simulink model "Demo_Intersection_cs"  (Simulink 7.6)
settings: Solver=FixedStepDiscrete  SolverMode=SingleTasking  StartTime=0.0  StopTime=13  FixedStep=1/20  RelTol=1e-3
PreLoadFcn:
  | check_NUTS_defined
  | model_closed = 0;
  | assignin('base',['model_closed_' bdroot],false);
InitFcn:
  | PreScanExperimentInitFcn(bdroot)
StopFcn:
  | PreScanExperimentStopFcn(bdroot);
  | 
undefined symbols (not defined in the file or in its folder): DiscIntNeverNeededParam
libraries: PreScanSimulinkLibrary x32, PreScanUsefulBlocks x8, simulink_extras x3
(part 2 of 5)

== system Demo_Intersection_cs/STATE_Toyota_Yaris_1 ==
  State : Inport  SampleTime=TimeStep
  Acceleration : Subsystem  mask(ToSensorWorld){PortName=Acceleration_Toyota_Yaris_1, PortIndex=21, PortWidth=3, TimeStep=1/20}
      mask prompts: PortName "Port Name [-]"; PortIndex "Index [-]"; PortWidth "Port Dimensions [-]"; TimeStep "Upload Period [s]"
      mask help: Sends signal(s) from Simulink to the Sensor World
      mask Help:
      | Sends signal(s) from Simulink to the Sensor World.
      | 
      | - Port Name [-]: specifies the name of the output terminal of the Simulink block.
      | - Index [-]: specifies the start position in the output vector sent to the Sensor World
      | - Port dimensions [-]: specifies the width (number of scalars) of the output port
      | - Upload period [s]: specifies the upload period (in seconds) of the port.
      mask Display: port_label('input', 1, PortName)
  Demux : Demux  Outputs=5
  Position : Subsystem  mask(ToSensorWorld){PortName=Position_Toyota_Yaris_1, PortIndex=15, PortWidth=3, TimeStep=1/20}
      mask prompts: PortName "Port Name [-]"; PortIndex "Index [-]"; PortWidth "Port Dimensions [-]"; TimeStep "Upload Period [s]"
      mask help: Sends signal(s) from Simulink to the Sensor World
      mask Help:
      | Sends signal(s) from Simulink to the Sensor World.
      | 
      | - Port Name [-]: specifies the name of the output terminal of the Simulink block.
      | - Index [-]: specifies the start position in the output vector sent to the Sensor World
      | - Port dimensions [-]: specifies the width (number of scalars) of the output port
      | - Upload period [s]: specifies the upload period (in seconds) of the port.
      mask Display: port_label('input', 1, PortName)
  RPY : Subsystem  mask(ToSensorWorld){PortName=RPY_Toyota_Yaris_1, PortIndex=24, PortWidth=3, TimeStep=1/20}
      mask prompts: PortName "Port Name [-]"; PortIndex "Index [-]"; PortWidth "Port Dimensions [-]"; TimeStep "Upload Period [s]"
      mask help: Sends signal(s) from Simulink to the Sensor World
      mask Help:
      | Sends signal(s) from Simulink to the Sensor World.
      | 
      | - Port Name [-]: specifies the name of the output terminal of the Simulink block.
      | - Index [-]: specifies the start position in the output vector sent to the Sensor World
      | - Port dimensions [-]: specifies the width (number of scalars) of the output port
      | - Upload period [s]: specifies the upload period (in seconds) of the port.
      mask Display: port_label('input', 1, PortName)
  Velocity : Subsystem  mask(ToSensorWorld){PortName=Velocity_Toyota_Yaris_1, PortIndex=18, PortWidth=3, TimeStep=1/20}
      mask prompts: PortName "Port Name [-]"; PortIndex "Index [-]"; PortWidth "Port Dimensions [-]"; TimeStep "Upload Period [s]"
      mask help: Sends signal(s) from Simulink to the Sensor World
      mask Help:
      | Sends signal(s) from Simulink to the Sensor World.
      | 
      | - Port Name [-]: specifies the name of the output terminal of the Simulink block.
      | - Index [-]: specifies the start position in the output vector sent to the Sensor World
      | - Port dimensions [-]: specifies the width (number of scalars) of the output port
      | - Upload period [s]: specifies the upload period (in seconds) of the port.
      mask Display: port_label('input', 1, PortName)
  iniBODYAngles wrtVEH [rad] : Constant  Value=[Roll0 Pitch0 0]  SampleTime=TimeStep
  iniVEHAngles wrtGLOB [rad] : Constant  Value=[0 0 Yaw0]  SampleTime=TimeStep
  iniVEHposition wrtGLOB [m] : Constant  Value=[x0 y0 z0]  SampleTime=TimeStep
  state2FullState : PreScanSimulinkLibrary/state2FullState  SystemSampleTime=-1
  velRPY : Subsystem  mask(ToSensorWorld){PortName=velRPY_Toyota_Yaris_1, PortIndex=27, PortWidth=3, TimeStep=1/20}
      mask prompts: PortName "Port Name [-]"; PortIndex "Index [-]"; PortWidth "Port Dimensions [-]"; TimeStep "Upload Period [s]"
      mask help: Sends signal(s) from Simulink to the Sensor World
      mask Help:
      | Sends signal(s) from Simulink to the Sensor World.
      | 
      | - Port Name [-]: specifies the name of the output terminal of the Simulink block.
      | - Index [-]: specifies the start position in the output vector sent to the Sensor World
      | - Port dimensions [-]: specifies the width (number of scalars) of the output port
      | - Upload period [s]: specifies the upload period (in seconds) of the port.
      mask Display: port_label('input', 1, PortName)
  wires:
  Demux/5 -> velRPY/1(Y)
  Demux/4 -> RPY/1(Y)
  Demux/3 -> Acceleration/1(Y)
  Demux/2 -> Velocity/1(Y)
  Demux/1 -> Position/1(Y)
  State/1 -> state2FullState/1
  state2FullState/1 -> Demux/1
  iniVEHposition wrtGLOB [m]/1 -> state2FullState/2
  iniBODYAngles wrtVEH [rad]/1 -> state2FullState/3
  iniVEHAngles wrtGLOB [rad]/1 -> state2FullState/4

== system Demo_Intersection_cs/SetActuators ==
  Bus Creator : BusCreator  Inputs=1
  Data Store Read : DataStoreRead  DataStoreName=SimCoreActuators  SampleTime=TimeStep
  SendActuators : M-S-Function  FunctionName=SendActuatorsBlock  Parameters=TimeStep NrOfActuators
  dummy : Outport
  tag scope: SimCoreInfo=global
  wires:
  Bus Creator/1 -> [SimCoreInfo]  "SimCore"
  SendActuators/2 -> Bus Creator/1  "ComputationTime[s]"
  SendActuators/1 -> dummy/1
  Data Store Read/1 -> SendActuators/1

== system Demo_Intersection_cs/SimCoreInfo ==
  Bus Selector : BusSelector  OutputSignals=ComputationTime[s]
  Time : Scope
      settings: TimeRange=10  YMin=0  YMax=0.5  SaveName=ComputationTime
  wires:
  Bus Selector/1 -> Time/1  "<ComputationTime[s]>"
  [SimCoreInfo] -> Bus Selector/1

== system Demo_Intersection_cs/Toyota_Previa_1 ==
  SELF_Toyota_Previa_1 : Inport  Tag=SELFInport
  Antenna_Tx_3_BusAssignment : BusAssignment  Tag=BusAntennaT  AssignedSignals=Intention
  Antenna_Tx_3_Mux : Subsystem  Tag=MuxAntennaT  mask(PreScan Mux Block:){Channel=1, TimeStep=1/20}
      mask prompts: TimeStep "Time Step [s]"
      settings: DeleteFcn=PreScanBlockDeleteFcn;
      mask Display:
      | fprintf('Channel: %d',Channel)
      | port_label('input', 1, 'Warning signal ID')
      | port_label('input', 2, 'Maneuvre ID')
      | port_label('input', 3, 'Vehicle Type')
      | port_label('input', 4, 'Braking Capacity')
      | port_label('input', 5, 'Vehicle Size')
      | port_label('input', 6, 'spare')
  Constant1 : Constant  Value=2
  Ground_{1..5} (5 alike) : Ground
  SELF_Demux : Subsystem  Tag=DemuxSELF
      settings: DeleteFcn=PreScanBlockDeleteFcn;
      mask Type: PreScan Demux Block:
      mask Display:
      | port_label('output',1,'x [m]')
      | port_label('output',2,'y [m]')
      | port_label('output',3,'z [m]','texmode','on')
      | port_label('output',4,'Rotx [deg]','texmode','on')
      | port_label('output',5,'Roty [deg]','texmode','on')
      | port_label('output',6,'Rotz [deg]','texmode','on')
      | port_label('output',7,'GPS lat [deg]','texmode','on')
      | port_label('output',8,'GPS long [deg]','texmode','on')
      | port_label('output',9,'GPS alt [m]','texmode','on')
      | port_label('output',10,'Velocity [m/s]')
      | port_label('output',11,'Heading [deg]')
      | port_label('output',12,'Yaw rate [deg/s]')
  Sum : Sum  Inputs=|++
  Terminator_{1..12} (12 alike) : Terminator
  Trajectories : Subsystem  Tag=Trajectories
      mask Display: image(imread('Trajectory.png'));
  STATE_Toyota_Previa_1 : Outport  Tag=StateOutport
  Antenna_Tx_3 : Outport  Tag=AntennaTOutport  Port=2
  wires:
  Constant1/1 -> Sum/2
  [Lane3_Intention] -> Sum/1
  SELF_Toyota_Previa_1/1 -> SELF_Demux/1(SELF)
  Antenna_Tx_3_Mux/2(Out2) -> [Antenna_Tx_3]
  [Antenna_Tx_3] -> Antenna_Tx_3_BusAssignment/1
  Antenna_Tx_3_BusAssignment/1 -> Antenna_Tx_3_Mux/6(spare)
  Antenna_Tx_3_Mux/1(Out1) -> Antenna_Tx_3/1
  Trajectories/1(State) -> STATE_Toyota_Previa_1/1
  Sum/1 -> Trajectories/1(In1)
  [Lane3_Intention] -> Antenna_Tx_3_BusAssignment/2
  Ground_1/1 -> Antenna_Tx_3_Mux/1(warning_signal_id)
  Ground_2/1 -> Antenna_Tx_3_Mux/2(maneuvre_id)
  Ground_3/1 -> Antenna_Tx_3_Mux/3(vehicle_type)
  Ground_4/1 -> Antenna_Tx_3_Mux/4(brakingcapacity)
  Ground_5/1 -> Antenna_Tx_3_Mux/5(vehicle_size)
  SELF_Demux/1(x [m]) -> Terminator_1/1
  SELF_Demux/2(y [m]) -> Terminator_2/1
  SELF_Demux/3(z [m]) -> Terminator_3/1
  SELF_Demux/4(rotx [deg]) -> Terminator_4/1
  SELF_Demux/5(roty [deg]) -> Terminator_5/1
  SELF_Demux/6(rotz [deg]) -> Terminator_6/1
  SELF_Demux/7(GPS lat [deg]) -> Terminator_7/1
  SELF_Demux/8(GPS long [deg]) -> Terminator_8/1
  SELF_Demux/9(GPS alt [m]) -> Terminator_9/1
  SELF_Demux/10(velocity [m/s]) -> Terminator_10/1
  SELF_Demux/11(heading [deg]) -> Terminator_11/1
  SELF_Demux/12(yaw rate [deg/s]) -> Terminator_12/1

== system Demo_Intersection_cs/Toyota_Yaris_1 ==
  SELF_Toyota_Yaris_1 : Inport  Tag=SELFInport
  Antenna_Tx_2_BusAssignment : BusAssignment  Tag=BusAntennaT  AssignedSignals=Intention
  Antenna_Tx_2_Mux : Subsystem  Tag=MuxAntennaT  mask(PreScan Mux Block:){Channel=1, TimeStep=1/20}
      mask prompts: TimeStep "Time Step [s]"
      settings: DeleteFcn=PreScanBlockDeleteFcn;
      mask Display:
      | fprintf('Channel: %d',Channel)
      | port_label('input', 1, 'Warning signal ID')
      | port_label('input', 2, 'Maneuvre ID')
      | port_label('input', 3, 'Vehicle Type')
      | port_label('input', 4, 'Braking Capacity')
      | port_label('input', 5, 'Vehicle Size')
      | port_label('input', 6, 'spare')
  Constant1 : Constant  Value=2
  Ground_{1..5} (5 alike) : Ground
  SELF_Demux : Subsystem  Tag=DemuxSELF
      settings: DeleteFcn=PreScanBlockDeleteFcn;
      mask Type: PreScan Demux Block:
      mask Display:
      | port_label('output',1,'x [m]')
      | port_label('output',2,'y [m]')
      | port_label('output',3,'z [m]','texmode','on')
      | port_label('output',4,'Rotx [deg]','texmode','on')
      | port_label('output',5,'Roty [deg]','texmode','on')
      | port_label('output',6,'Rotz [deg]','texmode','on')
      | port_label('output',7,'GPS lat [deg]','texmode','on')
      | port_label('output',8,'GPS long [deg]','texmode','on')
      | port_label('output',9,'GPS alt [m]','texmode','on')
      | port_label('output',10,'Velocity [m/s]')
      | port_label('output',11,'Heading [deg]')
      | port_label('output',12,'Yaw rate [deg/s]')
  Sum : Sum  Inputs=|++
  Terminator_{1..12} (12 alike) : Terminator
  Trajectories : Subsystem  Tag=Trajectories
      mask Display: image(imread('Trajectory.png'));
  STATE_Toyota_Yaris_1 : Outport  Tag=StateOutport
  Antenna_Tx_2 : Outport  Tag=AntennaTOutport  Port=2
  wires:
  Constant1/1 -> Sum/2
  [Lane2_Intention] -> Sum/1
  SELF_Toyota_Yaris_1/1 -> SELF_Demux/1(SELF)
  Antenna_Tx_2_Mux/2(Out2) -> [Antenna_Tx_2]
  [Antenna_Tx_2] -> Antenna_Tx_2_BusAssignment/1
  Antenna_Tx_2_BusAssignment/1 -> Antenna_Tx_2_Mux/6(spare)
  Antenna_Tx_2_Mux/1(Out1) -> Antenna_Tx_2/1
  Trajectories/1(State) -> STATE_Toyota_Yaris_1/1
  Sum/1 -> Trajectories/1(In1)
  [Lane2_Intention] -> Antenna_Tx_2_BusAssignment/2
  Ground_1/1 -> Antenna_Tx_2_Mux/1(warning_signal_id)
  Ground_2/1 -> Antenna_Tx_2_Mux/2(maneuvre_id)
  Ground_3/1 -> Antenna_Tx_2_Mux/3(vehicle_type)
  Ground_4/1 -> Antenna_Tx_2_Mux/4(brakingcapacity)
  Ground_5/1 -> Antenna_Tx_2_Mux/5(vehicle_size)
  SELF_Demux/1(x [m]) -> Terminator_1/1
  SELF_Demux/2(y [m]) -> Terminator_2/1
  SELF_Demux/3(z [m]) -> Terminator_3/1
  SELF_Demux/4(rotx [deg]) -> Terminator_4/1
  SELF_Demux/5(roty [deg]) -> Terminator_5/1
  SELF_Demux/6(rotz [deg]) -> Terminator_6/1
  SELF_Demux/7(GPS lat [deg]) -> Terminator_7/1
  SELF_Demux/8(GPS long [deg]) -> Terminator_8/1
  SELF_Demux/9(GPS alt [m]) -> Terminator_9/1
  SELF_Demux/10(velocity [m/s]) -> Terminator_10/1
  SELF_Demux/11(heading [deg]) -> Terminator_11/1
  SELF_Demux/12(yaw rate [deg/s]) -> Terminator_12/1

== system Demo_Intersection_cs/Mazda_RX8_1/Antenna_Rx_1_Demux ==
  AntennaR : Inport
  Bus Creator : BusCreator  Inputs=200
  Demux : Demux  Outputs=228
  Demux1 : Demux  Outputs=3
  Mux : Mux  Inputs=3
  Reorder : Subsystem  mask(Output reorder block){NrOfOutputs=228, NrOfObjects=3}
      mask prompts: NrOfOutputs "Number Of Outputs [-]"; NrOfObjects "Number Of Objects [-]"
      mask help: Change output order from object based to output type based
      mask init:
      | InputPortWidth=NrOfObjects*NrOfOutputs;
      | Input=1:InputPortWidth;
      | ReshapedInput=reshape(Input,NrOfOutputs,NrOfObjects);
      | TransposedReshapedInput=transpose(ReshapedInput);
      | Elements=reshape(TransposedReshapedInput,length(Input),1);
  Terminator_{9..12,17..18,20..23,25..30} (16 alike) : Terminator
  compas converter : Subsystem
  xyz2GPS : PreScanUsefulBlocks/xyz2GPS  CoordinateCount=3  GPS_base=[0.000000 0.000000 0.000]
  Vehicle_ID : Outport
  GPS_pos_lat_[deg] : Outport  Port=2
  GPS_pos_long_[deg] : Outport  Port=3
  GPS_pos_alt_[m] : Outport  Port=4
  Velocity_[m/s] : Outport  Port=5
  Acceleration_[m/s2] : Outport  Port=6
  Heading [deg] : Outport  Port=7
  warning_signal_id : Outport  Port=8
  maneuvre_id : Outport  Port=9
  vehicle_type : Outport  Port=10
  brakingcapacity : Outport  Port=11
  vehicle_size : Outport  Port=12
  spare : Outport  Port=13
  wires:
  Bus Creator/1 -> spare/1
  compas converter/1(heading [deg]) -> Heading [deg]/1
  Demux/1 -> Vehicle_ID/1
  Demux/2 -> Terminator_9/1
  Demux/3 -> Terminator_10/1
  Demux/4 -> Terminator_11/1
  Demux/5 -> Terminator_12/1
  Demux/6 -> Mux/1  "pos_x"
  Demux/7 -> Mux/2  "pos_y"
  Demux/8 -> Mux/3  "pos_z"
  Demux/10 -> Terminator_17/1
  Demux/11 -> Terminator_18/1
  Demux/12 -> Acceleration_[m/s2]/1
  Demux/13 -> Terminator_20/1
  Demux/14 -> Terminator_21/1
  Demux/15 -> Terminator_22/1
  Demux/16 -> Terminator_23/1
  Demux/17 -> compas converter/1(rotz [rad])
  Demux/18 -> Terminator_25/1
  Demux/19 -> Terminator_26/1
  Demux/20 -> Terminator_27/1
  Demux/21 -> Terminator_28/1
  Demux/22 -> Terminator_29/1
  Demux/23 -> Terminator_30/1
  Demux/9 -> Velocity_[m/s]/1
  Demux/24 -> warning_signal_id/1
  Demux/25 -> maneuvre_id/1
  Demux/26 -> vehicle_type/1
  Demux/27 -> brakingcapacity/1
  Demux/28 -> vehicle_size/1
  xyz2GPS/1 -> Demux1/1
  Demux1/1 -> GPS_pos_lat_[deg]/1
  Demux1/2 -> GPS_pos_long_[deg]/1
  Demux1/3 -> GPS_pos_alt_[m]/1
  Mux/1 -> xyz2GPS/1
  Reorder/1(Out) -> Demux/1
  AntennaR/1 -> Reorder/1(In)
  Demux/29 -> Bus Creator/1  "Intention"
  Demux/30 -> Bus Creator/2  "spare_2"
  Demux/31 -> Bus Creator/3  "spare_3"
  Demux/32 -> Bus Creator/4  "spare_4"
  Demux/33 -> Bus Creator/5  "spare_5"
  Demux/34 -> Bus Creator/6  "spare_6"
  Demux/35 -> Bus Creator/7  "spare_7"
  Demux/36 -> Bus Creator/8  "spare_8"
  Demux/37 -> Bus Creator/9  "spare_9"
  Demux/38 -> Bus Creator/10  "spare_10"
  Demux/39 -> Bus Creator/11  "spare_11"
  Demux/40 -> Bus Creator/12  "spare_12"
  Demux/41 -> Bus Creator/13  "spare_13"
  Demux/42 -> Bus Creator/14  "spare_14"
  Demux/43 -> Bus Creator/15  "spare_15"
  Demux/44 -> Bus Creator/16  "spare_16"
  Demux/45 -> Bus Creator/17  "spare_17"
  Demux/46 -> Bus Creator/18  "spare_18"
  Demux/47 -> Bus Creator/19  "spare_19"
  Demux/48 -> Bus Creator/20  "spare_20"
  Demux/49 -> Bus Creator/21  "spare_21"
  Demux/50 -> Bus Creator/22  "spare_22"
  Demux/51 -> Bus Creator/23  "spare_23"
  Demux/52 -> Bus Creator/24  "spare_24"
  Demux/53 -> Bus Creator/25  "spare_25"
  Demux/54 -> Bus Creator/26  "spare_26"
  Demux/55 -> Bus Creator/27  "spare_27"
  Demux/56 -> Bus Creator/28  "spare_28"
  Demux/57 -> Bus Creator/29  "spare_29"
  Demux/58 -> Bus Creator/30  "spare_30"
  Demux/59 -> Bus Creator/31  "spare_31"
  Demux/60 -> Bus Creator/32  "spare_32"
  Demux/61 -> Bus Creator/33  "spare_33"
  Demux/62 -> Bus Creator/34  "spare_34"
  Demux/63 -> Bus Creator/35  "spare_35"
  Demux/64 -> Bus Creator/36  "spare_36"
  Demux/65 -> Bus Creator/37  "spare_37"
  Demux/66 -> Bus Creator/38  "spare_38"
  Demux/67 -> Bus Creator/39  "spare_39"
  Demux/68 -> Bus Creator/40  "spare_40"
  Demux/69 -> Bus Creator/41  "spare_41"
  Demux/70 -> Bus Creator/42  "spare_42"
  Demux/71 -> Bus Creator/43  "spare_43"
  Demux/72 -> Bus Creator/44  "spare_44"
  Demux/73 -> Bus Creator/45  "spare_45"
  Demux/74 -> Bus Creator/46  "spare_46"
  Demux/75 -> Bus Creator/47  "spare_47"
  Demux/76 -> Bus Creator/48  "spare_48"
  Demux/77 -> Bus Creator/49  "spare_49"
  Demux/78 -> Bus Creator/50  "spare_50"
  Demux/79 -> Bus Creator/51  "spare_51"
  Demux/80 -> Bus Creator/52  "spare_52"
  Demux/81 -> Bus Creator/53  "spare_53"
  Demux/82 -> Bus Creator/54  "spare_54"
  Demux/83 -> Bus Creator/55  "spare_55"
  Demux/84 -> Bus Creator/56  "spare_56"
  Demux/85 -> Bus Creator/57  "spare_57"
  Demux/86 -> Bus Creator/58  "spare_58"
  Demux/87 -> Bus Creator/59  "spare_59"
  Demux/88 -> Bus Creator/60  "spare_60"
  Demux/89 -> Bus Creator/61  "spare_61"
  Demux/90 -> Bus Creator/62  "spare_62"
  Demux/91 -> Bus Creator/63  "spare_63"
  Demux/92 -> Bus Creator/64  "spare_64"
  Demux/93 -> Bus Creator/65  "spare_65"
  Demux/94 -> Bus Creator/66  "spare_66"
  Demux/95 -> Bus Creator/67  "spare_67"
  Demux/96 -> Bus Creator/68  "spare_68"
  Demux/97 -> Bus Creator/69  "spare_69"
  Demux/98 -> Bus Creator/70  "spare_70"
  Demux/99 -> Bus Creator/71  "spare_71"
  Demux/100 -> Bus Creator/72  "spare_72"
  Demux/101 -> Bus Creator/73  "spare_73"
  Demux/102 -> Bus Creator/74  "spare_74"
  Demux/103 -> Bus Creator/75  "spare_75"
  Demux/104 -> Bus Creator/76  "spare_76"
  Demux/105 -> Bus Creator/77  "spare_77"
  Demux/106 -> Bus Creator/78  "spare_78"
  Demux/107 -> Bus Creator/79  "spare_79"
  Demux/108 -> Bus Creator/80  "spare_80"
  Demux/109 -> Bus Creator/81  "spare_81"
  Demux/110 -> Bus Creator/82  "spare_82"
  Demux/111 -> Bus Creator/83  "spare_83"
  Demux/112 -> Bus Creator/84  "spare_84"
  Demux/113 -> Bus Creator/85  "spare_85"
  Demux/114 -> Bus Creator/86  "spare_86"
  Demux/115 -> Bus Creator/87  "spare_87"
  Demux/116 -> Bus Creator/88  "spare_88"
  Demux/117 -> Bus Creator/89  "spare_89"
  Demux/118 -> Bus Creator/90  "spare_90"
  Demux/119 -> Bus Creator/91  "spare_91"
  Demux/120 -> Bus Creator/92  "spare_92"
  Demux/121 -> Bus Creator/93  "spare_93"
  Demux/122 -> Bus Creator/94  "spare_94"
  Demux/123 -> Bus Creator/95  "spare_95"
  Demux/124 -> Bus Creator/96  "spare_96"
  Demux/125 -> Bus Creator/97  "spare_97"
  Demux/126 -> Bus Creator/98  "spare_98"
  Demux/127 -> Bus Creator/99  "spare_99"
  Demux/128 -> Bus Creator/100  "spare_100"
  Demux/129 -> Bus Creator/101  "spare_101"
  Demux/130 -> Bus Creator/102  "spare_102"
  Demux/131 -> Bus Creator/103  "spare_103"
  Demux/132 -> Bus Creator/104  "spare_104"
  Demux/133 -> Bus Creator/105  "spare_105"
  Demux/134 -> Bus Creator/106  "spare_106"
  Demux/135 -> Bus Creator/107  "spare_107"
  Demux/136 -> Bus Creator/108  "spare_108"
  Demux/137 -> Bus Creator/109  "spare_109"
  Demux/138 -> Bus Creator/110  "spare_110"
  Demux/139 -> Bus Creator/111  "spare_111"
  Demux/140 -> Bus Creator/112  "spare_112"
  Demux/141 -> Bus Creator/113  "spare_113"
  Demux/142 -> Bus Creator/114  "spare_114"
  Demux/143 -> Bus Creator/115  "spare_115"
  Demux/144 -> Bus Creator/116  "spare_116"
  Demux/145 -> Bus Creator/117  "spare_117"
  Demux/146 -> Bus Creator/118  "spare_118"
  Demux/147 -> Bus Creator/119  "spare_119"
  Demux/148 -> Bus Creator/120  "spare_120"
  Demux/149 -> Bus Creator/121  "spare_121"
  Demux/150 -> Bus Creator/122  "spare_122"
  Demux/151 -> Bus Creator/123  "spare_123"
  Demux/152 -> Bus Creator/124  "spare_124"
  Demux/153 -> Bus Creator/125  "spare_125"
  Demux/154 -> Bus Creator/126  "spare_126"
  Demux/155 -> Bus Creator/127  "spare_127"
  Demux/156 -> Bus Creator/128  "spare_128"
  Demux/157 -> Bus Creator/129  "spare_129"
  Demux/158 -> Bus Creator/130  "spare_130"
  Demux/159 -> Bus Creator/131  "spare_131"
  Demux/160 -> Bus Creator/132  "spare_132"
  Demux/161 -> Bus Creator/133  "spare_133"
  Demux/162 -> Bus Creator/134  "spare_134"
  Demux/163 -> Bus Creator/135  "spare_135"
  Demux/164 -> Bus Creator/136  "spare_136"
  Demux/165 -> Bus Creator/137  "spare_137"
  Demux/166 -> Bus Creator/138  "spare_138"
  Demux/167 -> Bus Creator/139  "spare_139"
  Demux/168 -> Bus Creator/140  "spare_140"
  Demux/169 -> Bus Creator/141  "spare_141"
  Demux/170 -> Bus Creator/142  "spare_142"
  Demux/171 -> Bus Creator/143  "spare_143"
  Demux/172 -> Bus Creator/144  "spare_144"
  Demux/173 -> Bus Creator/145  "spare_145"
  Demux/174 -> Bus Creator/146  "spare_146"
  Demux/175 -> Bus Creator/147  "spare_147"
  Demux/176 -> Bus Creator/148  "spare_148"
  Demux/177 -> Bus Creator/149  "spare_149"
  Demux/178 -> Bus Creator/150  "spare_150"
  Demux/179 -> Bus Creator/151  "spare_151"
  Demux/180 -> Bus Creator/152  "spare_152"
  Demux/181 -> Bus Creator/153  "spare_153"
  Demux/182 -> Bus Creator/154  "spare_154"
  Demux/183 -> Bus Creator/155  "spare_155"
  Demux/184 -> Bus Creator/156  "spare_156"
  Demux/185 -> Bus Creator/157  "spare_157"
  Demux/186 -> Bus Creator/158  "spare_158"
  Demux/187 -> Bus Creator/159  "spare_159"
  Demux/188 -> Bus Creator/160  "spare_160"
  Demux/189 -> Bus Creator/161  "spare_161"
  Demux/190 -> Bus Creator/162  "spare_162"
  Demux/191 -> Bus Creator/163  "spare_163"
  Demux/192 -> Bus Creator/164  "spare_164"
  Demux/193 -> Bus Creator/165  "spare_165"
  Demux/194 -> Bus Creator/166  "spare_166"
  Demux/195 -> Bus Creator/167  "spare_167"
  Demux/196 -> Bus Creator/168  "spare_168"
  Demux/197 -> Bus Creator/169  "spare_169"
  Demux/198 -> Bus Creator/170  "spare_170"
  Demux/199 -> Bus Creator/171  "spare_171"
  Demux/200 -> Bus Creator/172  "spare_172"
  Demux/201 -> Bus Creator/173  "spare_173"
  Demux/202 -> Bus Creator/174  "spare_174"
  Demux/203 -> Bus Creator/175  "spare_175"
  Demux/204 -> Bus Creator/176  "spare_176"
  Demux/205 -> Bus Creator/177  "spare_177"
  Demux/206 -> Bus Creator/178  "spare_178"
  Demux/207 -> Bus Creator/179  "spare_179"
  Demux/208 -> Bus Creator/180  "spare_180"
  Demux/209 -> Bus Creator/181  "spare_181"
  Demux/210 -> Bus Creator/182  "spare_182"
  Demux/211 -> Bus Creator/183  "spare_183"
  Demux/212 -> Bus Creator/184  "spare_184"
  Demux/213 -> Bus Creator/185  "spare_185"
  Demux/214 -> Bus Creator/186  "spare_186"
  Demux/215 -> Bus Creator/187  "spare_187"
  Demux/216 -> Bus Creator/188  "spare_188"
  Demux/217 -> Bus Creator/189  "spare_189"
  Demux/218 -> Bus Creator/190  "spare_190"
  Demux/219 -> Bus Creator/191  "spare_191"
  Demux/220 -> Bus Creator/192  "spare_192"
  Demux/221 -> Bus Creator/193  "spare_193"
  Demux/222 -> Bus Creator/194  "spare_194"
  Demux/223 -> Bus Creator/195  "spare_195"
  Demux/224 -> Bus Creator/196  "spare_196"
  Demux/225 -> Bus Creator/197  "spare_197"
  Demux/226 -> Bus Creator/198  "spare_198"
  Demux/227 -> Bus Creator/199  "spare_199"
  Demux/228 -> Bus Creator/200  "spare_200"

== system Demo_Intersection_cs/Mazda_RX8_1/Dynamics_Empty ==
  note: For state mode 'Dynamic' positions
      | are not taken into account, as they
      | are computed by integrating velocity.
      | Click annotation for Help.
  Ground_{1..9} (9 alike) : Ground
  MuxState : Subsystem  Tag=MuxState  mask{positioningmode=off, TimeStep=1/20}
      mask prompts: positioningmode "Positioning Mode"; TimeStep "Auto Assigned: Time Step [s]"
      settings: DeleteFcn=PreScanBlockDeleteFcn;
  State : Outport  Tag=StateOutport
  wires:
  MuxState/1(state) -> State/1
  Ground_1/1 -> MuxState/1(x [m])
  Ground_2/1 -> MuxState/2(y [m])
  Ground_3/1 -> MuxState/3(z [m])
  Ground_4/1 -> MuxState/4(dx [m/s])
  Ground_5/1 -> MuxState/5(dy [m/s])
  Ground_6/1 -> MuxState/6(dz [m/s])
  Ground_7/1 -> MuxState/7(R [rad])
  Ground_8/1 -> MuxState/8(P [rad])
  Ground_9/1 -> MuxState/9(Y [rad])

== system Demo_Intersection_cs/Mazda_RX8_1/Retreive car data using ID info ==
  note: id=3
  note: id=4
  note: id=5
  note: id=3
  note: id=4
  note: id=5
  note: id=3
  note: id=4
  note: id=5
  note: id=3
  note: id=4
  note: id=5
  note: id=3
  note: id=4
  note: id=5
  note: Assumption:
      | All vehicles are visible all time.
      | So the data can be ordered by using the id order.
      | id=0 (meaning no detection) does not exist
  note: id=5
  note: id=3
  note: id=4
  note: id=3
  note: id=4
  note: id=5
  Lat_detected : Inport
  Lon_detected : Inport  Port=2
  Alt_detected : Inport  Port=3
  Intention_detected : Inport  Port=4
  Heading_detected : Inport  Port=5
  Complex to Magnitude-Angle1 : ComplexToMagnitudeAngle
  Complex to Magnitude-Angle2 : ComplexToMagnitudeAngle
  Complex to Magnitude-Angle3 : ComplexToMagnitudeAngle
  Demux{,4..7} (5 alike) : Demux  Outputs=3
  Demux1 : Demux  Outputs=2
  Demux2 : Demux  Outputs=2
  Demux3 : Demux  Outputs=2
  GPS2xyz : PreScanUsefulBlocks/GPS2xyz  CoordinateCount=1  GPS_base=[0 0 0]
  GPS2xyz1 : PreScanUsefulBlocks/GPS2xyz  CoordinateCount=1  GPS_base=[0 0 0]
  GPS2xyz2 : PreScanUsefulBlocks/GPS2xyz  CoordinateCount=1  GPS_base=[0 0 0]
  Mux : Mux
  Mux1 : Mux
  Mux2 : Mux
  Mux3 : Mux  Inputs=3
  Mux4 : Mux  Inputs=3
  Mux5 : Mux  Inputs=3
  Radians to Degrees : simulink_extras/Transformations/Radians to Degrees  SystemSampleTime=-1
  Radians to Degrees1 : simulink_extras/Transformations/Radians to Degrees  SystemSampleTime=-1
  Radians to Degrees2 : simulink_extras/Transformations/Radians to Degrees  SystemSampleTime=-1
  Real-Imag to Complex1 : RealImagToComplex
  Real-Imag to Complex2 : RealImagToComplex
  Real-Imag to Complex3 : RealImagToComplex
  Selector : Selector  IndexOptions=Index vector (dialog)  Indices=[1 2]  OutputSizes=1
  Selector1 : Selector  IndexOptions=Index vector (dialog)  Indices=[1 2]  OutputSizes=1
  Selector2 : Selector  IndexOptions=Index vector (dialog)  Indices=[1 2]  OutputSizes=1
  Cabstar : Outport
  Yaris : Outport  Port=2
  Previa : Outport  Port=3
  wires:
  GPS2xyz/1 -> Selector/1
  Selector/1 -> Demux1/1
  Selector1/1 -> Demux2/1
  Intention_detected/1 -> Demux/1
  Demux/1 -> Mux/3  "intention"
  Demux/2 -> Mux1/3  "intention"
  Demux/3 -> Mux2/3  "intention"
  Mux/1 -> Yaris/1
  Mux1/1 -> Cabstar/1
  Mux2/1 -> Previa/1
  Complex to Magnitude-Angle1/1 -> Mux/1  "range"
  Radians to Degrees/1 -> Mux/2  "angle"
  Complex to Magnitude-Angle1/2 -> Radians to Degrees/1
  Real-Imag to Complex1/1 -> Complex to Magnitude-Angle1/1
  Demux1/1 -> Real-Imag to Complex1/1
  Demux1/2 -> Real-Imag to Complex1/2
  Complex to Magnitude-Angle2/1 -> Mux1/1  "range"
  Radians to Degrees1/1 -> Mux1/2  "angle"
  Complex to Magnitude-Angle2/2 -> Radians to Degrees1/1
  Real-Imag to Complex2/1 -> Complex to Magnitude-Angle2/1
  Demux2/1 -> Real-Imag to Complex2/1
  Demux2/2 -> Real-Imag to Complex2/2
  Selector2/1 -> Demux3/1
  Complex to Magnitude-Angle3/1 -> Mux2/1  "range"
  Radians to Degrees2/1 -> Mux2/2  "angle"
  Complex to Magnitude-Angle3/2 -> Radians to Degrees2/1
  Real-Imag to Complex3/1 -> Complex to Magnitude-Angle3/1
  Demux3/1 -> Real-Imag to Complex3/1
  Demux3/2 -> Real-Imag to Complex3/2
  GPS2xyz1/1 -> Selector1/1
  GPS2xyz2/1 -> Selector2/1
  Lat_detected/1 -> Demux5/1
  Alt_detected/1 -> Demux7/1
  Lon_detected/1 -> Demux6/1
  Demux5/1 -> Mux3/1
  Demux5/2 -> Mux4/1
  Demux5/3 -> Mux5/1
  Demux6/1 -> Mux3/2
  Demux6/2 -> Mux4/2
  Demux7/1 -> Mux3/3
  Demux6/3 -> Mux5/2
  Demux7/2 -> Mux4/3
  Demux7/3 -> Mux5/3
  Mux5/1 -> GPS2xyz2/1
  Mux4/1 -> GPS2xyz1/1
  Mux3/1 -> GPS2xyz/1
  Heading_detected/1 -> Demux4/1
  Demux4/1 -> Mux/4  "heading"
  Demux4/2 -> Mux1/4  "heading"
  Demux4/3 -> Mux2/4  "heading"

== system Demo_Intersection_cs/Mazda_RX8_1/SELF_Demux ==
  SELF : Inport
  Demux1 : Demux  Outputs=3
  Demux2 : Demux  Outputs=3
  Demux3 : Demux  Outputs=[3 3 1 1]
  Demux4 : Demux  Outputs=3
  Gain : Gain  Gain=180/pi
  Gain1 : Gain  Gain=180/pi
  Selector : Selector  InputPortWidth=3  IndexOptions=Index vector (dialog)  Indices=[3]  OutputSizes=1
  compas converter : Subsystem
  xyz2GPS : PreScanUsefulBlocks/xyz2GPS  CoordinateCount=1  GPS_base=[0.000000 0.000000 0.000]
  x [m] : Outport
  y [m] : Outport  Port=2
  z [m] : Outport  Port=3
  rotx [deg] : Outport  Port=4
  roty [deg] : Outport  Port=5
  rotz [deg] : Outport  Port=6
  GPS lat [deg] : Outport  Port=7
  GPS long [deg] : Outport  Port=8
  GPS alt [m] : Outport  Port=9
  velocity [m/s] : Outport  Port=10
  heading [deg] : Outport  Port=11
  yaw rate [deg/s] : Outport  Port=12
  wires:
  Demux3/4 -> Gain1/1
  Gain1/1 -> yaw rate [deg/s]/1
  Demux3/3 -> velocity [m/s]/1
  compas converter/1(heading [deg]) -> heading [deg]/1
  xyz2GPS/1 -> Demux4/1
  Demux4/3 -> GPS alt [m]/1
  Demux4/2 -> GPS long [deg]/1
  Demux4/1 -> GPS lat [deg]/1
  Demux3/2 -> Gain/1, Selector/1
  Demux3/1 -> xyz2GPS/1, Demux1/1
  SELF/1 -> Demux3/1
  Demux2/3 -> rotz [deg]/1
  Demux2/2 -> roty [deg]/1
  Demux2/1 -> rotx [deg]/1
  Demux1/3 -> z [m]/1
  Demux1/2 -> y [m]/1
  Demux1/1 -> x [m]/1
  Gain/1 -> Demux2/1
  Selector/1 -> compas converter/1(rotz [rad])

== system Demo_Intersection_cs/Mazda_RX8_1/Sort AIR Output based on ID ==
  In6 : Inport
  In1 : Inport  Port=2
  In2 : Inport  Port=3
  In3 : Inport  Port=4
  In4 : Inport  Port=5
  In5 : Inport  Port=6
  Constant1 : Constant  Value=mode
  Constant2 : Constant  Value=ignorezero
  Embedded MATLAB Function : Stateflow chart  TreatAsAtomicUnit=on
  Selector{1..5} (5 alike) : Selector  IndexOptions=Index vector (port)  Indices=[1 3]  OutputSizes=1
  Out1 : Outport
  Out2 : Outport  Port=2
  Out3 : Outport  Port=3
  Out5 : Outport  Port=4
  Out4 : Outport  Port=5
  wires:
  Constant2/1 -> Embedded MATLAB Function/3(ignorezero)
  Constant1/1 -> Embedded MATLAB Function/2(mode)
  In6/1 -> Embedded MATLAB Function/1(u)
  In4/1 -> Selector4/1
  In3/1 -> Selector3/1
  In2/1 -> Selector2/1
  Selector4/1 -> Out4/1
  Selector3/1 -> Out3/1
  Selector2/1 -> Out2/1
  Selector1/1 -> Out1/1
  In1/1 -> Selector1/1
  Embedded MATLAB Function/1(y) -> Selector3/2, Selector4/2, Selector5/2, Selector2/2, Selector1/2
  In5/1 -> Selector5/1, Embedded MATLAB Function/4(ids)
  Selector5/1 -> Out5/1

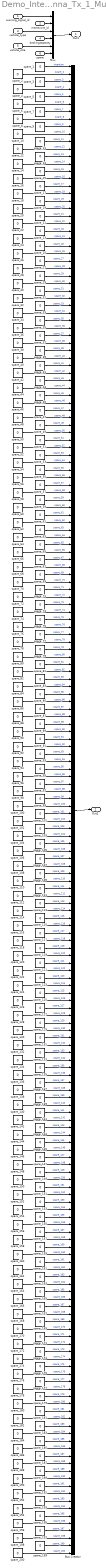
== system Demo_Intersection_cs/Nissan_Cabstar_1/Antenna_Tx_1_Mux ==
  warning_signal_id : Inport  SampleTime=TimeStep
  maneuvre_id : Inport  Port=2  SampleTime=TimeStep
  vehicle_type : Inport  Port=3  SampleTime=TimeStep
  brakingcapacity : Inport  Port=4  SampleTime=TimeStep
  vehicle_size : Inport  Port=5  SampleTime=TimeStep
  spare : Inport  Port=6  SampleTime=TimeStep
  Bus Creator : BusCreator  Inputs=200
  Mux : Mux  Inputs=6
  spare_{1..200} (200 alike) : Constant  Value=0  SampleTime=TimeStep
  Out1 : Outport
  Out2 : Outport  Port=2  SampleTime=TimeStep
  wires:
  spare_200/1 -> Bus Creator/200  "spare_200"
  spare_199/1 -> Bus Creator/199  "spare_199"
  spare_198/1 -> Bus Creator/198  "spare_198"
  spare_197/1 -> Bus Creator/197  "spare_197"
  spare_196/1 -> Bus Creator/196  "spare_196"
  spare_195/1 -> Bus Creator/195  "spare_195"
  spare_194/1 -> Bus Creator/194  "spare_194"
  spare_193/1 -> Bus Creator/193  "spare_193"
  spare_192/1 -> Bus Creator/192  "spare_192"
  spare_191/1 -> Bus Creator/191  "spare_191"
  spare_190/1 -> Bus Creator/190  "spare_190"
  spare_189/1 -> Bus Creator/189  "spare_189"
  spare_188/1 -> Bus Creator/188  "spare_188"
  spare_187/1 -> Bus Creator/187  "spare_187"
  spare_186/1 -> Bus Creator/186  "spare_186"
  spare_185/1 -> Bus Creator/185  "spare_185"
  spare_184/1 -> Bus Creator/184  "spare_184"
  spare_183/1 -> Bus Creator/183  "spare_183"
  spare_182/1 -> Bus Creator/182  "spare_182"
  spare_181/1 -> Bus Creator/181  "spare_181"
  spare_180/1 -> Bus Creator/180  "spare_180"
  spare_179/1 -> Bus Creator/179  "spare_179"
  spare_178/1 -> Bus Creator/178  "spare_178"
  spare_177/1 -> Bus Creator/177  "spare_177"
  spare_176/1 -> Bus Creator/176  "spare_176"
  spare_175/1 -> Bus Creator/175  "spare_175"
  spare_174/1 -> Bus Creator/174  "spare_174"
  spare_173/1 -> Bus Creator/173  "spare_173"
  spare_172/1 -> Bus Creator/172  "spare_172"
  spare_171/1 -> Bus Creator/171  "spare_171"
  spare_170/1 -> Bus Creator/170  "spare_170"
  spare_169/1 -> Bus Creator/169  "spare_169"
  spare_168/1 -> Bus Creator/168  "spare_168"
  spare_167/1 -> Bus Creator/167  "spare_167"
  spare_166/1 -> Bus Creator/166  "spare_166"
  spare_165/1 -> Bus Creator/165  "spare_165"
  spare_164/1 -> Bus Creator/164  "spare_164"
  spare_163/1 -> Bus Creator/163  "spare_163"
  spare_162/1 -> Bus Creator/162  "spare_162"
  spare_161/1 -> Bus Creator/161  "spare_161"
  spare_160/1 -> Bus Creator/160  "spare_160"
  spare_159/1 -> Bus Creator/159  "spare_159"
  spare_158/1 -> Bus Creator/158  "spare_158"
  spare_157/1 -> Bus Creator/157  "spare_157"
  spare_156/1 -> Bus Creator/156  "spare_156"
  spare_155/1 -> Bus Creator/155  "spare_155"
  spare_154/1 -> Bus Creator/154  "spare_154"
  spare_153/1 -> Bus Creator/153  "spare_153"
  spare_152/1 -> Bus Creator/152  "spare_152"
  spare_151/1 -> Bus Creator/151  "spare_151"
  spare_150/1 -> Bus Creator/150  "spare_150"
  spare_149/1 -> Bus Creator/149  "spare_149"
  spare_148/1 -> Bus Creator/148  "spare_148"
  spare_147/1 -> Bus Creator/147  "spare_147"
  spare_146/1 -> Bus Creator/146  "spare_146"
  spare_145/1 -> Bus Creator/145  "spare_145"
  spare_144/1 -> Bus Creator/144  "spare_144"
  spare_143/1 -> Bus Creator/143  "spare_143"
  spare_142/1 -> Bus Creator/142  "spare_142"
  spare_141/1 -> Bus Creator/141  "spare_141"
  spare_140/1 -> Bus Creator/140  "spare_140"
  spare_139/1 -> Bus Creator/139  "spare_139"
  spare_138/1 -> Bus Creator/138  "spare_138"
  spare_137/1 -> Bus Creator/137  "spare_137"
  spare_136/1 -> Bus Creator/136  "spare_136"
  spare_135/1 -> Bus Creator/135  "spare_135"
  spare_134/1 -> Bus Creator/134  "spare_134"
  spare_133/1 -> Bus Creator/133  "spare_133"
  spare_132/1 -> Bus Creator/132  "spare_132"
  spare_131/1 -> Bus Creator/131  "spare_131"
  spare_130/1 -> Bus Creator/130  "spare_130"
  spare_129/1 -> Bus Creator/129  "spare_129"
  spare_128/1 -> Bus Creator/128  "spare_128"
  spare_127/1 -> Bus Creator/127  "spare_127"
  spare_126/1 -> Bus Creator/126  "spare_126"
  spare_125/1 -> Bus Creator/125  "spare_125"
  spare_124/1 -> Bus Creator/124  "spare_124"
  spare_123/1 -> Bus Creator/123  "spare_123"
  spare_122/1 -> Bus Creator/122  "spare_122"
  spare_121/1 -> Bus Creator/121  "spare_121"
  spare_120/1 -> Bus Creator/120  "spare_120"
  spare_119/1 -> Bus Creator/119  "spare_119"
  spare_118/1 -> Bus Creator/118  "spare_118"
  spare_117/1 -> Bus Creator/117  "spare_117"
  spare_116/1 -> Bus Creator/116  "spare_116"
  spare_115/1 -> Bus Creator/115  "spare_115"
  spare_114/1 -> Bus Creator/114  "spare_114"
  spare_113/1 -> Bus Creator/113  "spare_113"
  spare_112/1 -> Bus Creator/112  "spare_112"
  spare_111/1 -> Bus Creator/111  "spare_111"
  spare_110/1 -> Bus Creator/110  "spare_110"
  spare_109/1 -> Bus Creator/109  "spare_109"
  spare_108/1 -> Bus Creator/108  "spare_108"
  spare_107/1 -> Bus Creator/107  "spare_107"
  spare_106/1 -> Bus Creator/106  "spare_106"
  spare_105/1 -> Bus Creator/105  "spare_105"
  spare_104/1 -> Bus Creator/104  "spare_104"
  spare_103/1 -> Bus Creator/103  "spare_103"
  spare_102/1 -> Bus Creator/102  "spare_102"
  spare_101/1 -> Bus Creator/101  "spare_101"
  spare_100/1 -> Bus Creator/100  "spare_100"
  spare_99/1 -> Bus Creator/99  "spare_99"
  spare_98/1 -> Bus Creator/98  "spare_98"
  spare_97/1 -> Bus Creator/97  "spare_97"
  spare_96/1 -> Bus Creator/96  "spare_96"
  spare_95/1 -> Bus Creator/95  "spare_95"
  spare_94/1 -> Bus Creator/94  "spare_94"
  spare_93/1 -> Bus Creator/93  "spare_93"
  spare_92/1 -> Bus Creator/92  "spare_92"
  spare_91/1 -> Bus Creator/91  "spare_91"
  spare_90/1 -> Bus Creator/90  "spare_90"
  spare_89/1 -> Bus Creator/89  "spare_89"
  spare_88/1 -> Bus Creator/88  "spare_88"
  spare_87/1 -> Bus Creator/87  "spare_87"
  spare_86/1 -> Bus Creator/86  "spare_86"
  spare_85/1 -> Bus Creator/85  "spare_85"
  spare_84/1 -> Bus Creator/84  "spare_84"
  spare_83/1 -> Bus Creator/83  "spare_83"
  spare_82/1 -> Bus Creator/82  "spare_82"
  spare_81/1 -> Bus Creator/81  "spare_81"
  spare_80/1 -> Bus Creator/80  "spare_80"
  spare_79/1 -> Bus Creator/79  "spare_79"
  spare_78/1 -> Bus Creator/78  "spare_78"
  spare_77/1 -> Bus Creator/77  "spare_77"
  spare_76/1 -> Bus Creator/76  "spare_76"
  spare_75/1 -> Bus Creator/75  "spare_75"
  spare_74/1 -> Bus Creator/74  "spare_74"
  spare_73/1 -> Bus Creator/73  "spare_73"
  spare_72/1 -> Bus Creator/72  "spare_72"
  spare_71/1 -> Bus Creator/71  "spare_71"
  spare_70/1 -> Bus Creator/70  "spare_70"
  spare_69/1 -> Bus Creator/69  "spare_69"
  spare_68/1 -> Bus Creator/68  "spare_68"
  spare_67/1 -> Bus Creator/67  "spare_67"
  spare_66/1 -> Bus Creator/66  "spare_66"
  spare_65/1 -> Bus Creator/65  "spare_65"
  spare_64/1 -> Bus Creator/64  "spare_64"
  spare_63/1 -> Bus Creator/63  "spare_63"
  spare_62/1 -> Bus Creator/62  "spare_62"
  spare_61/1 -> Bus Creator/61  "spare_61"
  spare_60/1 -> Bus Creator/60  "spare_60"
  spare_59/1 -> Bus Creator/59  "spare_59"
  spare_58/1 -> Bus Creator/58  "spare_58"
  spare_57/1 -> Bus Creator/57  "spare_57"
  spare_56/1 -> Bus Creator/56  "spare_56"
  spare_55/1 -> Bus Creator/55  "spare_55"
  spare_54/1 -> Bus Creator/54  "spare_54"
  spare_53/1 -> Bus Creator/53  "spare_53"
  spare_52/1 -> Bus Creator/52  "spare_52"
  spare_51/1 -> Bus Creator/51  "spare_51"
  spare_50/1 -> Bus Creator/50  "spare_50"
  spare_49/1 -> Bus Creator/49  "spare_49"
  spare_48/1 -> Bus Creator/48  "spare_48"
  spare_47/1 -> Bus Creator/47  "spare_47"
  spare_46/1 -> Bus Creator/46  "spare_46"
  spare_45/1 -> Bus Creator/45  "spare_45"
  spare_44/1 -> Bus Creator/44  "spare_44"
  spare_43/1 -> Bus Creator/43  "spare_43"
  spare_42/1 -> Bus Creator/42  "spare_42"
  spare_41/1 -> Bus Creator/41  "spare_41"
  spare_40/1 -> Bus Creator/40  "spare_40"
  spare_39/1 -> Bus Creator/39  "spare_39"
  spare_38/1 -> Bus Creator/38  "spare_38"
  spare_37/1 -> Bus Creator/37  "spare_37"
  spare_36/1 -> Bus Creator/36  "spare_36"
  spare_35/1 -> Bus Creator/35  "spare_35"
  spare_34/1 -> Bus Creator/34  "spare_34"
  spare_33/1 -> Bus Creator/33  "spare_33"
  spare_32/1 -> Bus Creator/32  "spare_32"
  spare_31/1 -> Bus Creator/31  "spare_31"
  spare_30/1 -> Bus Creator/30  "spare_30"
  spare_29/1 -> Bus Creator/29  "spare_29"
  spare_28/1 -> Bus Creator/28  "spare_28"
  spare_27/1 -> Bus Creator/27  "spare_27"
  spare_26/1 -> Bus Creator/26  "spare_26"
  spare_25/1 -> Bus Creator/25  "spare_25"
  spare_24/1 -> Bus Creator/24  "spare_24"
  spare_23/1 -> Bus Creator/23  "spare_23"
  spare_22/1 -> Bus Creator/22  "spare_22"
  spare_21/1 -> Bus Creator/21  "spare_21"
  spare_19/1 -> Bus Creator/19  "spare_19"
  spare_18/1 -> Bus Creator/18  "spare_18"
  spare_17/1 -> Bus Creator/17  "spare_17"
  spare_16/1 -> Bus Creator/16  "spare_16"
  spare_15/1 -> Bus Creator/15  "spare_15"
  spare_14/1 -> Bus Creator/14  "spare_14"
  spare_13/1 -> Bus Creator/13  "spare_13"
  spare_12/1 -> Bus Creator/12  "spare_12"
  spare_11/1 -> Bus Creator/11  "spare_11"
  spare_10/1 -> Bus Creator/10  "spare_10"
  spare_9/1 -> Bus Creator/9  "spare_9"
  spare_8/1 -> Bus Creator/8  "spare_8"
  spare_7/1 -> Bus Creator/7  "spare_7"
  spare_6/1 -> Bus Creator/6  "spare_6"
  spare_5/1 -> Bus Creator/5  "spare_5"
  spare_4/1 -> Bus Creator/4  "spare_4"
  spare_3/1 -> Bus Creator/3  "spare_3"
  spare_2/1 -> Bus Creator/2  "spare_2"
  warning_signal_id/1 -> Mux/1
  maneuvre_id/1 -> Mux/2
  vehicle_type/1 -> Mux/3
  brakingcapacity/1 -> Mux/4
  vehicle_size/1 -> Mux/5
  Mux/1 -> Out1/1
  Bus Creator/1 -> Out2/1
  spare/1 -> Mux/6
  spare_1/1 -> Bus Creator/1  "Intention"
  spare_20/1 -> Bus Creator/20  "spare_20"

== system Demo_Intersection_cs/Nissan_Cabstar_1/SELF_Demux ==
  SELF : Inport
  Demux1 : Demux  Outputs=3
  Demux2 : Demux  Outputs=3
  Demux3 : Demux  Outputs=[3 3 1 1]
  Demux4 : Demux  Outputs=3
  Gain : Gain  Gain=180/pi
  Gain1 : Gain  Gain=180/pi
  Selector : Selector  InputPortWidth=3  IndexOptions=Index vector (dialog)  Indices=[3]  OutputSizes=1
  compas converter : Subsystem
  xyz2GPS : PreScanUsefulBlocks/xyz2GPS  CoordinateCount=1  GPS_base=[0.000000 0.000000 0.000]
  x [m] : Outport
  y [m] : Outport  Port=2
  z [m] : Outport  Port=3
  rotx [deg] : Outport  Port=4
  roty [deg] : Outport  Port=5
  rotz [deg] : Outport  Port=6
  GPS lat [deg] : Outport  Port=7
  GPS long [deg] : Outport  Port=8
  GPS alt [m] : Outport  Port=9
  velocity [m/s] : Outport  Port=10
  heading [deg] : Outport  Port=11
  yaw rate [deg/s] : Outport  Port=12
  wires:
  Demux3/4 -> Gain1/1
  Gain1/1 -> yaw rate [deg/s]/1
  Demux3/3 -> velocity [m/s]/1
  compas converter/1(heading [deg]) -> heading [deg]/1
  xyz2GPS/1 -> Demux4/1
  Demux4/3 -> GPS alt [m]/1
  Demux4/2 -> GPS long [deg]/1
  Demux4/1 -> GPS lat [deg]/1
  Demux3/2 -> Gain/1, Selector/1
  Demux3/1 -> xyz2GPS/1, Demux1/1
  SELF/1 -> Demux3/1
  Demux2/3 -> rotz [deg]/1
  Demux2/2 -> roty [deg]/1
  Demux2/1 -> rotx [deg]/1
  Demux1/3 -> z [m]/1
  Demux1/2 -> y [m]/1
  Demux1/1 -> x [m]/1
  Gain/1 -> Demux2/1
  Selector/1 -> compas converter/1(rotz [rad])

== system Demo_Intersection_cs/Nissan_Cabstar_1/Trajectories ==
  SelectTraj1 : Inport
  PathFollowerSva_1 : Subsystem  Tag=Trajectory  mask(PreScan Source Block: Trajectory){FileName='PathFollowerSva_1.mat', TimeStep=1/20}
      mask prompts: TimeStep "Time Step [s]"
      mask help:
      | The Trajectory block contains the trajectories defined in the PreScan Experiment Editor. The output of the trajectory block is the (vehicle) State.
      |
      | For more information, please click Help.
      mask init:
      | [direc,name]=fileparts(get_param(bdroot, 'FileName'));
      | load([direc,'/Trajectories/',FileName])
      | trajectory=trajectory';
      | 
      | traj.time=trajectory(:,1);%[];
      | traj.signals.values=trajectory(:,2:19);
      | traj.dimensions=18;
      | traj.label='';
      | 
      | SampleTime=traj.time(2)-traj.time(1);
      settings: DeleteFcn=PreScanBlockDeleteFcn;
      mask Help: eval('openHelp(312)')
      mask Display: fprintf(FileName)
  PathFollowerSva_1_Offset : Constant  Tag=TrajectoryOffset  Value="[0  0  0  0  0  0]"
  PathFollowerSva_2 : Subsystem  Tag=Trajectory  mask(PreScan Source Block: Trajectory){FileName='PathFollowerSva_2.mat', TimeStep=1/20}
      mask prompts: TimeStep "Time Step [s]"
      mask help:
      | The Trajectory block contains the trajectories defined in the PreScan Experiment Editor. The output of the trajectory block is the (vehicle) State.
      |
      | For more information, please click Help.
      mask init: same as Demo_Intersection_cs/Nissan_Cabstar_1/Trajectories/PathFollowerSva_1
      settings: DeleteFcn=PreScanBlockDeleteFcn;
      mask Help: eval('openHelp(312)')
      mask Display: fprintf(FileName)
  PathFollowerSva_2_Offset : Constant  Tag=TrajectoryOffset  Value="[0  0  0  0  0  0]"
  PathFollowerSva_3 : Subsystem  Tag=Trajectory  mask(PreScan Source Block: Trajectory){FileName='PathFollowerSva_3.mat', TimeStep=1/20}
      mask prompts: TimeStep "Time Step [s]"
      mask help:
      | The Trajectory block contains the trajectories defined in the PreScan Experiment Editor. The output of the trajectory block is the (vehicle) State.
      |
      | For more information, please click Help.
      mask init: same as Demo_Intersection_cs/Nissan_Cabstar_1/Trajectories/PathFollowerSva_1
      settings: DeleteFcn=PreScanBlockDeleteFcn;
      mask Help: eval('openHelp(312)')
      mask Display: fprintf(FileName)
  PathFollowerSva_3_Offset : Constant  Tag=TrajectoryOffset  Value="[0  0  0  0  0  0]"
  SelectTraj : Constant  Tag=TrajSelector
  Switch : MultiPortSwitch  Tag=TrajSwitch  zeroidx=off
  Terminator_1 : Terminator
  Traj2State1 : Subsystem  Tag=Traj2State
      settings: DeleteFcn=PreScanBlockDeleteFcn;
      mask Type: PreScan Demux Block:
  Traj2State2 : Subsystem  Tag=Traj2State
      settings: DeleteFcn=PreScanBlockDeleteFcn;
      mask Type: PreScan Demux Block:
  Traj2State3 : Subsystem  Tag=Traj2State
      settings: DeleteFcn=PreScanBlockDeleteFcn;
      mask Type: PreScan Demux Block:
  State : Outport  Tag=TrajOutport
  wires:
  PathFollowerSva_1/1(trajectory) -> Traj2State1/1(Traj Org)
  PathFollowerSva_1_Offset/1 -> Traj2State1/2(Offset)
  Traj2State1/1(state) -> Switch/2
  PathFollowerSva_2/1(trajectory) -> Traj2State2/1(Traj Org)
  PathFollowerSva_2_Offset/1 -> Traj2State2/2(Offset)
  Traj2State2/1(state) -> Switch/3
  PathFollowerSva_3/1(trajectory) -> Traj2State3/1(Traj Org)
  PathFollowerSva_3_Offset/1 -> Traj2State3/2(Offset)
  Traj2State3/1(state) -> Switch/4
  Switch/1 -> State/1
  SelectTraj1/1 -> Switch/1
  SelectTraj/1 -> Terminator_1/1

== system Demo_Intersection_cs/STATE_Mazda_RX8_1/Acceleration ==
  Y : Inport
  Assignment : Assignment  IndexMode=Zero-based  SampleTime=TimeStep  IndexOptions=Starting index (dialog)  Indices=PortIndex  OutputSizes=[1 1]
  Data Store Read : DataStoreRead  DataStoreName=SimCoreActuators  SampleTime=TimeStep
  Data Store Write : DataStoreWrite  DataStoreName=SimCoreActuators
  wires:
  Assignment/1 -> Data Store Write/1
  Data Store Read/1 -> Assignment/1
  Y/1 -> Assignment/2

== system Demo_Intersection_cs/STATE_Mazda_RX8_1/Position ==
  Y : Inport
  Assignment : Assignment  IndexMode=Zero-based  SampleTime=TimeStep  IndexOptions=Starting index (dialog)  Indices=PortIndex  OutputSizes=[1 1]
  Data Store Read : DataStoreRead  DataStoreName=SimCoreActuators  SampleTime=TimeStep
  Data Store Write : DataStoreWrite  DataStoreName=SimCoreActuators
  wires:
  Y/1 -> Assignment/2
  Data Store Read/1 -> Assignment/1
  Assignment/1 -> Data Store Write/1

== system Demo_Intersection_cs/STATE_Mazda_RX8_1/RPY ==
  Y : Inport
  Assignment : Assignment  IndexMode=Zero-based  SampleTime=TimeStep  IndexOptions=Starting index (dialog)  Indices=PortIndex  OutputSizes=[1 1]
  Data Store Read : DataStoreRead  DataStoreName=SimCoreActuators  SampleTime=TimeStep
  Data Store Write : DataStoreWrite  DataStoreName=SimCoreActuators
  wires:
  Assignment/1 -> Data Store Write/1
  Data Store Read/1 -> Assignment/1
  Y/1 -> Assignment/2

== system Demo_Intersection_cs/STATE_Mazda_RX8_1/Velocity ==
  Y : Inport
  Assignment : Assignment  IndexMode=Zero-based  SampleTime=TimeStep  IndexOptions=Starting index (dialog)  Indices=PortIndex  OutputSizes=[1 1]
  Data Store Read : DataStoreRead  DataStoreName=SimCoreActuators  SampleTime=TimeStep
  Data Store Write : DataStoreWrite  DataStoreName=SimCoreActuators
  wires:
  Assignment/1 -> Data Store Write/1
  Data Store Read/1 -> Assignment/1
  Y/1 -> Assignment/2

== system Demo_Intersection_cs/STATE_Mazda_RX8_1/velRPY ==
  Y : Inport
  Assignment : Assignment  IndexMode=Zero-based  SampleTime=TimeStep  IndexOptions=Starting index (dialog)  Indices=PortIndex  OutputSizes=[1 1]
  Data Store Read : DataStoreRead  DataStoreName=SimCoreActuators  SampleTime=TimeStep
  Data Store Write : DataStoreWrite  DataStoreName=SimCoreActuators
  wires:
  Assignment/1 -> Data Store Write/1
  Data Store Read/1 -> Assignment/1
  Y/1 -> Assignment/2

== system Demo_Intersection_cs/STATE_Nissan_Cabstar_1/Acceleration ==
  Y : Inport
  Assignment : Assignment  IndexMode=Zero-based  SampleTime=TimeStep  IndexOptions=Starting index (dialog)  Indices=PortIndex  OutputSizes=[1 1]
  Data Store Read : DataStoreRead  DataStoreName=SimCoreActuators  SampleTime=TimeStep
  Data Store Write : DataStoreWrite  DataStoreName=SimCoreActuators
  wires:
  Assignment/1 -> Data Store Write/1
  Data Store Read/1 -> Assignment/1
  Y/1 -> Assignment/2

== system Demo_Intersection_cs/STATE_Nissan_Cabstar_1/Position ==
  Y : Inport
  Assignment : Assignment  IndexMode=Zero-based  SampleTime=TimeStep  IndexOptions=Starting index (dialog)  Indices=PortIndex  OutputSizes=[1 1]
  Data Store Read : DataStoreRead  DataStoreName=SimCoreActuators  SampleTime=TimeStep
  Data Store Write : DataStoreWrite  DataStoreName=SimCoreActuators
  wires:
  Y/1 -> Assignment/2
  Data Store Read/1 -> Assignment/1
  Assignment/1 -> Data Store Write/1

== system Demo_Intersection_cs/STATE_Nissan_Cabstar_1/RPY ==
  Y : Inport
  Assignment : Assignment  IndexMode=Zero-based  SampleTime=TimeStep  IndexOptions=Starting index (dialog)  Indices=PortIndex  OutputSizes=[1 1]
  Data Store Read : DataStoreRead  DataStoreName=SimCoreActuators  SampleTime=TimeStep
  Data Store Write : DataStoreWrite  DataStoreName=SimCoreActuators
  wires:
  Assignment/1 -> Data Store Write/1
  Data Store Read/1 -> Assignment/1
  Y/1 -> Assignment/2
